simulink model "highway_designer_sim2020a"  (R2020a)
settings: Solver=FixedStepAuto  StartTime=0.0  StopTime=10.0  RelTol=1e-3
model workspace (MAT data in the model file):
  firstWarning = 1
  originalScenarioChecksum = 'FFC6E04D7DC672EFDEEDFE7D709B94D3'
libraries: drivingscenarioandsensors x5, sim3dprobsensorlib x3, sim3dautolib x3, sim3dlib x1
settings Model: Creator=joann  LastModifiedBy=joann

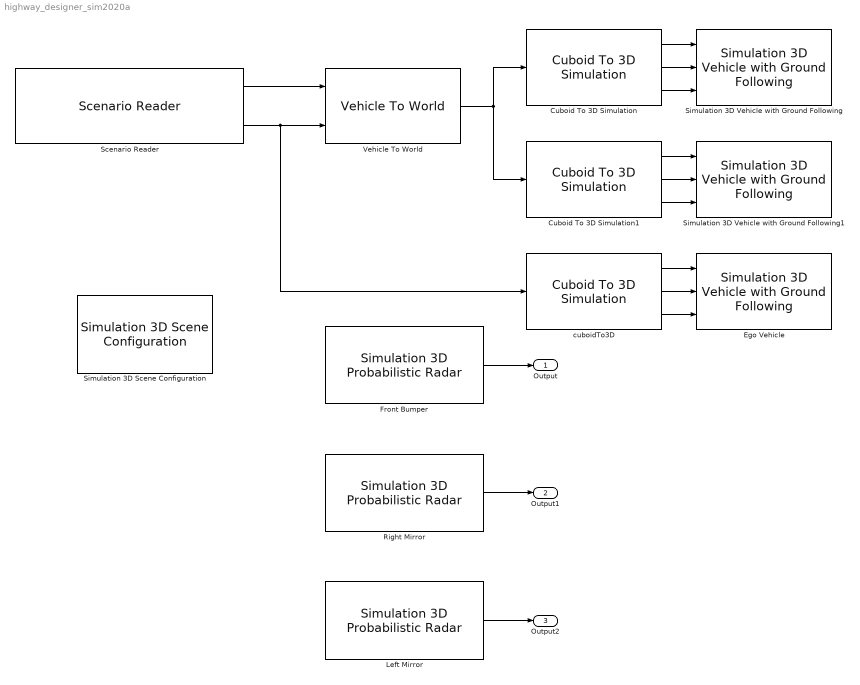
== system highway_designer_sim2020a ==
  " Left Mirror" : sim3dprobsensorlib/Simulation 3D Probabilistic Radar  Priority=1  sensorTag=Sim3dSensor3  sensorId=3  sensorName=Sim3dSensor3  vehTagList={'Ego Vehicle';'Scene Origin';'SimulinkVehicle1';'SimulinkVehicle2'}  vehTag=Ego Vehicle  mountLoc=Left mirror  offsetFlag=off  tmountOffset=[0, 0, 0]  rmountOffset=[0, 0, 0]  AzimuthResolution=4  ElevationResolution=10  RangeResolution=2.5  RangeRateResolution=0.5  AzimuthBiasFraction=0.1  ElevationBiasFraction=0.1  RangeBiasFraction=0.05  RangeRateBiasFraction=0.05  FieldOfView=[ 20, 5 ]  DetectionRange=[ 1, 150 ]  RangeRateLimits=[ -100, 100 ]  DetectionProbability=0.9  FalseAlarmRate=1e-6  ReferenceRange=100  ReferenceRCS=0  HasElevation=on  HasRangeRate=on  HasNoise=on  HasFalseAlarms=on  InitialSeedSource=Repeatable  InitialSeed=0  MaxNumDetections=50  DetectionCoordinates=Ego Cartesian  SpecifyOutputBusName=off  BusName=BusSimulation3DRadarTruthSensor  SampleTime=-1  mountPoint=[0.430000007152557 -1.08000004291534 1]  mountOrientation=[0 -90 0]  aMode=3  ID=3
      settings: SourceProductBaseCode=DR,VE
  Cuboid To 3D Simulation : drivingscenarioandsensors/Cuboid To 3D Simulation  SpecifyActorID=on  ActorIDToConvert=1  SimulateUsing=Interpreted execution
      settings: SourceProductBaseCode=DR
  Cuboid To 3D Simulation1 : drivingscenarioandsensors/Cuboid To 3D Simulation  SpecifyActorID=on  ActorIDToConvert=2  SimulateUsing=Interpreted execution
      settings: SourceProductBaseCode=DR
  Ego Vehicle : sim3dautolib/Simulation 3D Vehicle with Ground Following  Priority=-1  PassVehMesh=Muscle car  VehColor=Red  InitialPos=[0, 0, 0]  InitialRot=[0, 0, 0]  ActorName=Ego Vehicle  SampleTime=0.1  ActorType=SimulinkVehicle  ID=C  aMode=3  ActorTag=Ego Vehicle  CoordinateScheme=ISO  TransformOutportEnabled=off
      settings: SourceProductBaseCode=DR,VE
  Front Bumper : sim3dprobsensorlib/Simulation 3D Probabilistic Radar  Priority=1  sensorTag=Sim3dSensor1  sensorId=1  sensorName=Sim3dSensor1  vehTagList={'Ego Vehicle';'Scene Origin';'SimulinkVehicle1';'SimulinkVehicle2'}  vehTag=Ego Vehicle  mountLoc=Front bumper  offsetFlag=off  tmountOffset=[0, 0, 0]  rmountOffset=[0, 0, 0]  AzimuthResolution=4  ElevationResolution=10  RangeResolution=2.5  RangeRateResolution=0.5  AzimuthBiasFraction=0.1  ElevationBiasFraction=0.1  RangeBiasFraction=0.05  RangeRateBiasFraction=0.05  FieldOfView=[ 20, 5 ]  DetectionRange=[ 1, 150 ]  RangeRateLimits=[ -100, 100 ]  DetectionProbability=0.9  FalseAlarmRate=1e-6  ReferenceRange=100  ReferenceRCS=0  HasElevation=on  HasRangeRate=on  HasNoise=on  HasFalseAlarms=on  InitialSeedSource=Repeatable  InitialSeed=0  MaxNumDetections=50  DetectionCoordinates=Ego Cartesian  SpecifyOutputBusName=off  BusName=BusSimulation3DRadarTruthSensor  SampleTime=-1  mountPoint=[2.47350001335144 0 0.439999997615814]  mountOrientation=[0 0 0]  aMode=3  ID=1
      settings: SourceProductBaseCode=DR,VE
  Right Mirror : sim3dprobsensorlib/Simulation 3D Probabilistic Radar  Priority=1  sensorTag=Sim3dSensor2  sensorId=2  sensorName=Sim3dSensor2  vehTagList={'Ego Vehicle';'Scene Origin';'SimulinkVehicle1';'SimulinkVehicle2'}  vehTag=Ego Vehicle  mountLoc=Right mirror  offsetFlag=off  tmountOffset=[0, 0, 0]  rmountOffset=[0, 0, 0]  AzimuthResolution=4  ElevationResolution=10  RangeResolution=2.5  RangeRateResolution=0.5  AzimuthBiasFraction=0.1  ElevationBiasFraction=0.1  RangeBiasFraction=0.05  RangeRateBiasFraction=0.05  FieldOfView=[ 20, 5 ]  DetectionRange=[ 1, 150 ]  RangeRateLimits=[ -100, 100 ]  DetectionProbability=0.9  FalseAlarmRate=1e-6  ReferenceRange=100  ReferenceRCS=0  HasElevation=on  HasRangeRate=on  HasNoise=on  HasFalseAlarms=on  InitialSeedSource=Repeatable  InitialSeed=0  MaxNumDetections=50  DetectionCoordinates=Ego Cartesian  SpecifyOutputBusName=off  BusName=BusSimulation3DRadarTruthSensor  SampleTime=-1  mountPoint=[0.430000007152557 1.08000004291534 1]  mountOrientation=[0 -90 0]  aMode=3  ID=2
      settings: SourceProductBaseCode=DR,VE
  Scenario Reader : drivingscenarioandsensors/Scenario Reader  ScenarioSource=From file  ScenarioFileName=D:\Co_op\UWAFT\3D_Simulation_Environment\highway_designer_sim.mat  ScenarioVariableName=scenario  OutputCoordinateSystem=Vehicle coordinates  EgoVehicleSource=Scenario  OrientVehiclesOnRoad=off  EgoVehicleActorID=1  OutputEgoVehiclePose=on  SampleTime=0.1  LaneBoundaryOutput=None  LaneBoundaryDistance=0:0.5:9.5  LaneBoundaryLocation=Center of lane markings  BusNameSource=Auto  BusName=BusActors  BusName2Source=Auto  BusName2=BusLaneBoundaries  BusName3Source=Auto  BusName3=BusEgoActor  ShowCoordinateLabels=on  SimulateUsing=Interpreted execution
  Simulation 3D Scene Configuration : sim3dlib/Simulation 3D Scene Configuration  Priority=0  ProjectFormat=Default Scenes  SceneDesc=Straight road  ProjectName=VehicleSimulation.exe  ScenePath=/Game/Maps/HwStrght  vehTagList={'Ego Vehicle';'Scene Origin';'SimulinkVehicle1';'SimulinkVehicle2'}  vehTag=Ego Vehicle  OpVisEn=off  Ts=0.1  EnableWindow=on  sensorTag=MainCamera1  sensorId=1  sensorName=MainCamera1  mountLoc=Origin  offsetFlag=off  tmountOffset=[0, 0, 0]  rmountOffset=[0, 0, 0]  HorizontalResolution=1280  VerticalResolution=720  HorizontalFOV=60  mountPoint=[0 0 0]  mountOrientation=[0 0 0]  aMode=3  ID=1
      settings: SourceProductBaseCode=DR,VE
  Simulation 3D Vehicle with Ground Following : sim3dautolib/Simulation 3D Vehicle with Ground Following  Priority=-1  PassVehMesh=Muscle car  VehColor=Red  InitialPos=[0, 0, 0]  InitialRot=[0, 0, 0]  ActorName=SimulinkVehicle1  SampleTime=0.1  ActorType=SimulinkVehicle  ID=1  aMode=3  ActorTag=SimulinkVehicle1  CoordinateScheme=ISO  TransformOutportEnabled=off
      settings: SourceProductBaseCode=DR,VE
  Simulation 3D Vehicle with Ground Following1 : sim3dautolib/Simulation 3D Vehicle with Ground Following  Priority=-1  PassVehMesh=Muscle car  VehColor=Red  InitialPos=[0, 0, 0]  InitialRot=[0, 0, 0]  ActorName=SimulinkVehicle2  SampleTime=0.1  ActorType=SimulinkVehicle  ID=2  aMode=3  ActorTag=SimulinkVehicle2  CoordinateScheme=ISO  TransformOutportEnabled=off
      settings: SourceProductBaseCode=DR,VE
  Vehicle To World : drivingscenarioandsensors/Vehicle To World  BusNameSource=Auto  BusName=BusVehicleToWorldActors  SimulateUsing=Interpreted execution
      settings: SourceProductBaseCode=DR
  cuboidTo3D : drivingscenarioandsensors/Cuboid To 3D Simulation  SpecifyActorID=on  ActorIDToConvert=3  SimulateUsing=Interpreted execution
      settings: SourceProductBaseCode=DR
  Output : Outport
  Output1 : Outport  Port=2
  Output2 : Outport  Port=3
  wires:
  Scenario Reader/1 -> Vehicle To World/1
  Scenario Reader/2 -> cuboidTo3D/1, Vehicle To World/2
  Vehicle To World/1 -> Cuboid To 3D Simulation/1, Cuboid To 3D Simulation1/1
  Cuboid To 3D Simulation/1 -> Simulation 3D Vehicle with Ground Following/1
  Cuboid To 3D Simulation/2 -> Simulation 3D Vehicle with Ground Following/2
  Cuboid To 3D Simulation/3 -> Simulation 3D Vehicle with Ground Following/3
  Cuboid To 3D Simulation1/1 -> Simulation 3D Vehicle with Ground Following1/1
  Cuboid To 3D Simulation1/2 -> Simulation 3D Vehicle with Ground Following1/2
  Cuboid To 3D Simulation1/3 -> Simulation 3D Vehicle with Ground Following1/3
  cuboidTo3D/1 -> Ego Vehicle/1
  cuboidTo3D/2 -> Ego Vehicle/2
  cuboidTo3D/3 -> Ego Vehicle/3
  Front Bumper/1 -> Output/1
  Right Mirror/1 -> Output1/1
  " Left Mirror"/1 -> Output2/1
